simulink model "TType_OffGrid_Inverter_5Step_7Step_SVPWM_THIPWM_Sim"  (R2022b)
settings: Solver=FixedStepDiscrete  StartTime=0.0  StopTime=1  FixedStep=1e-6  RelTol=1e-3
undefined symbols (not defined in the file): L1
libraries: spsSeriesRLCBranchLib x14, spsMosfetLib x12, spsRMSLib x3, simulink x3, spsVoltageMeasurementLib x3, spsThreePhaseVIMeasurementLib x2, spsDCVoltageSourceLib x1, spsGroundLib x1, spsPower3phInstantaneousLib x1, spspowerguiLib x1
settings Model: Creator=XIAO  LastModifiedBy=XIAO
settings SolverCC: AutoInsertRateTranBlk=on
settings DataIOCC: ReturnWorkspaceOutputs=off

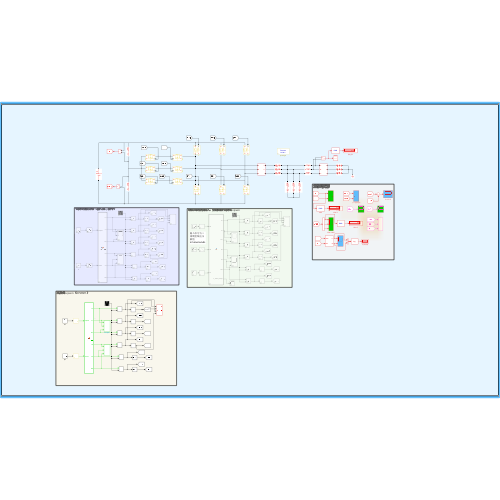
[thumbnail: Simulink's stored preview of the top-level diagram]
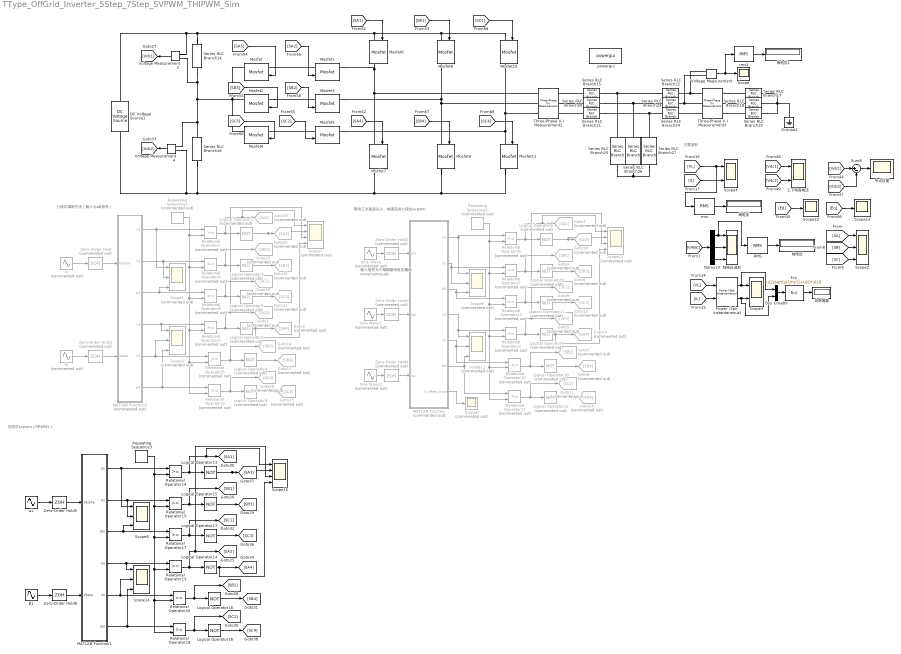
== system TType_OffGrid_Inverter_5Step_7Step_SVPWM_THIPWM_Sim ==
  note: 五段式svpwm（DPWM1）
  note: 输入信号为三相期望线电压幅值
      | m=uinvmx/udc
  note: 等效三次谐波注入，快速完成七段式svpwm
  note: 七段式调制方法（输入为αβ信号）
  note: 主要波形
  Bus Creator : BusCreator  Inputs=2
  DC Voltage Source1 : spsDCVoltageSourceLib/DC Voltage Source  Amplitude=60  Measurements=None
  Demux3 : Demux  Outputs=3
  Fcn : Fcn  Expr=u(1)/sqrt(u(1)*u(1)+u(2)*u(2))
  Goto1 : Goto  Commented=on  GotoTag=SA2
  Goto10 : Goto  Commented=on  GotoTag=SA4
  Goto11 : Goto  Commented=on  GotoTag=SC2
  Goto12 : Goto  Commented=on  GotoTag=SC3
  Goto13 : Goto  Commented=on  GotoTag=SB1
  Goto14 : Goto  Commented=on  GotoTag=SB2
  Goto15 : Goto  Commented=on  GotoTag=SB3
  Goto16 : Goto  Commented=on  GotoTag=SA1
  Goto17 : Goto  Commented=on  GotoTag=SB4
  Goto18 : Goto  Commented=on  GotoTag=SC1
  Goto19 : Goto  Commented=on  GotoTag=SA3
  Goto2 : Goto  Commented=on  GotoTag=SA4
  Goto20 : Goto  Commented=on  GotoTag=SC2
  Goto21 : Goto  Commented=on  GotoTag=SC3
  Goto22 : Goto  Commented=on  GotoTag=SA3
  Goto23 : Goto  Commented=on  GotoTag=SC4
  Goto24 : Goto  Commented=on  GotoTag=SC4
  Goto3 : Goto  Commented=on  GotoTag=SA2
  Goto4 : Goto  Commented=on  GotoTag=SB1
  Goto5 : Goto  Commented=on  GotoTag=SB2
  Goto6 : Goto  Commented=on  GotoTag=SB3
  Goto7 : Goto  Commented=on  GotoTag=SA1
  Goto8 : Goto  Commented=on  GotoTag=SB4
  Goto9 : Goto  Commented=on  GotoTag=SC1
  Ground2 : spsGroundLib/Ground  LConnTagsString=a
  Logical Operator{1..12} (12 alike) : Logic  Commented=on  Operator=NOT  AllPortsSameDT=off  OutDataTypeStr=boolean
  Logical Operator{13..18} (6 alike) : Logic  Operator=NOT  AllPortsSameDT=off  OutDataTypeStr=boolean
  MATLAB Function : MATLAB Function  Commented=on  TreatAsAtomicUnit=on
  MATLAB Function1 : MATLAB Function  TreatAsAtomicUnit=on
  MATLAB Function2 : MATLAB Function  Commented=on  TreatAsAtomicUnit=on
  Mosfet{,1..11} (12 alike) : spsMosfetLib/Mosfet  Ron=0.1  Lon=0  Rd=0.01  Vfd=0  IC=0  Rs=1e5  Cs=inf  Measurements=on
  "Power (3ph, Instantaneous)" : spsPower3phInstantaneousLib/Power (3ph, Instantaneous)
  RMS : spsRMSLib/RMS  TrueRMS=on  Freq=50  RMSInit=120  Ts=1e-6
  Relational Operator{1..12} (12 alike) : RelationalOperator  Commented=on  OutDataTypeStr=boolean  RndMeth=Simplest  InputSameDT=off
  Relational Operator{13..18} (6 alike) : RelationalOperator  OutDataTypeStr=boolean  RndMeth=Simplest  InputSameDT=off
  Repeating Sequence1 : simulink/Sources/Repeating Sequence  Commented=on  rep_seq_t="[0  5e-5  1e-4]"  rep_seq_y=[0 8500 0]
  Repeating Sequence2 : simulink/Sources/Repeating Sequence  Commented=on  rep_seq_t="[0  5e-5  1e-4]"  rep_seq_y=[0 8500 0]
  Repeating Sequence3 : simulink/Sources/Repeating Sequence  rep_seq_t="[0  5e-5  1e-4]"  rep_seq_y=[0 8500 0]
  Scope : Scope
  Scope{1,5,9,11} (4 alike) : Scope  Commented=on  NumInputPorts=3
  Scope10 : Scope
  Scope12 : Scope  Commented=on  NumInputPorts=4
  Scope13 : Scope
  Scope14 : Scope  NumInputPorts=3
  Scope15 : Scope  NumInputPorts=4
  Scope2 : Scope  NumInputPorts=3
  Scope3 : Scope  NumInputPorts=2
  Scope4 : Scope  NumInputPorts=2
  Scope6 : Scope  Commented=on
  Scope7 : Scope  Commented=on  NumInputPorts=4
  Scope8 : Scope  NumInputPorts=3
  Series RLC Branch14 : spsSeriesRLCBranchLib/Series RLC Branch  LConnTagsString=__new0  RConnTagsString=__new0  BranchType=RC  Resistance=0.001  Inductance=1e-3  SetiL0=off  InitialCurrent=0  Capacitance=1000e-6  Setx0=off  InitialVoltage=260  Measurements=None
  Series RLC Branch15 : spsSeriesRLCBranchLib/Series RLC Branch  LConnTagsString=__new0  RConnTagsString=__new0  BranchType=RL  Resistance=1e-3  Inductance=2e-3  SetiL0=off  InitialCurrent=0  Capacitance=5.6e-3  Setx0=off  InitialVoltage=0  Measurements=None
  Series RLC Branch16 : spsSeriesRLCBranchLib/Series RLC Branch  LConnTagsString=__new0  RConnTagsString=__new0  BranchType=RC  Resistance=0.001  Inductance=1e-3  SetiL0=off  InitialCurrent=0  Capacitance=1000e-6  Setx0=off  InitialVoltage=200  Measurements=None
  Series RLC Branch17 : spsSeriesRLCBranchLib/Series RLC Branch  LConnTagsString=__new0  RConnTagsString=__new0  BranchType=RLC  Resistance=200  Inductance=0  SetiL0=off  InitialCurrent=0  Capacitance=0  Setx0=off  InitialVoltage=0  Measurements=None
  Series RLC Branch18 : spsSeriesRLCBranchLib/Series RLC Branch  LConnTagsString=__new0  RConnTagsString=__new0  BranchType=RLC  Resistance=200  Inductance=0  SetiL0=off  InitialCurrent=0  Capacitance=0  Setx0=off  InitialVoltage=0  Measurements=None
  Series RLC Branch19 : spsSeriesRLCBranchLib/Series RLC Branch  LConnTagsString=__new0  RConnTagsString=__new0  BranchType=RLC  Resistance=200  Inductance=0  SetiL0=off  InitialCurrent=0  Capacitance=0  Setx0=off  InitialVoltage=0  Measurements=None
  Series RLC Branch20 : spsSeriesRLCBranchLib/Series RLC Branch  LConnTagsString=__new0  RConnTagsString=__new0  BranchType=RL  Resistance=1e-3  Inductance=2e-3  SetiL0=off  InitialCurrent=0  Capacitance=5.6e-3  Setx0=off  InitialVoltage=0  Measurements=None
  Series RLC Branch21 : spsSeriesRLCBranchLib/Series RLC Branch  LConnTagsString=__new0  RConnTagsString=__new0  BranchType=RL  Resistance=1e-3  Inductance=2e-3  SetiL0=off  InitialCurrent=0  Capacitance=5.6e-3  Setx0=off  InitialVoltage=0  Measurements=None
  Series RLC Branch22 : spsSeriesRLCBranchLib/Series RLC Branch  LConnTagsString=__new0  RConnTagsString=__new0  BranchType=L  Resistance=1e-6  Inductance=1.5e-3  SetiL0=off  InitialCurrent=0  Capacitance=5.6e-3  Setx0=off  InitialVoltage=0  Measurements=None
  Series RLC Branch23 : spsSeriesRLCBranchLib/Series RLC Branch  LConnTagsString=__new0  RConnTagsString=__new0  BranchType=L  Resistance=1e-6  Inductance=1.5e-3  SetiL0=off  InitialCurrent=0  Capacitance=5.6e-3  Setx0=off  InitialVoltage=0  Measurements=None
  Series RLC Branch24 : spsSeriesRLCBranchLib/Series RLC Branch  LConnTagsString=__new0  RConnTagsString=__new0  BranchType=L  Resistance=1e-6  Inductance=1.5e-3  SetiL0=off  InitialCurrent=0  Capacitance=5.6e-3  Setx0=off  InitialVoltage=0  Measurements=None
  Series RLC Branch25 : spsSeriesRLCBranchLib/Series RLC Branch  LConnTagsString=__new0  RConnTagsString=__new0  BranchType=RC  Resistance=3  Inductance=L1  SetiL0=off  InitialCurrent=0  Capacitance=10.5e-6  Setx0=off  InitialVoltage=0  Measurements=None
  Series RLC Branch26 : spsSeriesRLCBranchLib/Series RLC Branch  LConnTagsString=__new0  RConnTagsString=__new0  BranchType=RC  Resistance=3  Inductance=L1  SetiL0=off  InitialCurrent=0  Capacitance=10.5e-6  Setx0=off  InitialVoltage=0  Measurements=None
  Series RLC Branch27 : spsSeriesRLCBranchLib/Series RLC Branch  LConnTagsString=__new0  RConnTagsString=__new0  BranchType=RC  Resistance=3  Inductance=L1  SetiL0=off  InitialCurrent=0  Capacitance=10.5e-6  Setx0=off  InitialVoltage=0  Measurements=None
  Sine Wave : Sin  Commented=on  Amplitude=0.7542  Frequency=2*pi*50  SampleTime=0
  Sine Wave1 : Sin  Commented=on  Amplitude=0.7542  Frequency=2*pi*50  Phase=2*pi/3  SampleTime=0
  Sine Wave2 : Sin  Commented=on  Amplitude=0.7542  Frequency=2*pi*50  Phase=-2*pi/3  SampleTime=0
  Sum8 : Sum  Inputs=|+-
  Three-Phase V-I Measurement2 : spsThreePhaseVIMeasurementLib/Three-Phase V-I Measurement  VoltageMeasurement=phase-to-phase  SetLabelV=on  LabelV=VABC  Vpu=off  VpuLL=off  CurrentMeasurement=yes  SetLabelI=on  LabelI=Iinv  Ipu=off  Pbase=100e6  Vbase=500e3  OutputType=Complex  PhasorSimulation=off  PSBequivalent=0
  Three-Phase V-I Measurement3 : spsThreePhaseVIMeasurementLib/Three-Phase V-I Measurement  VoltageMeasurement=phase-to-ground  SetLabelV=on  LabelV=VL  Vpu=off  VpuLL=off  CurrentMeasurement=yes  SetLabelI=on  LabelI=IL  Ipu=off  Pbase=100e6  Vbase=500e3  OutputType=Complex  PhasorSimulation=off  PSBequivalent=0
  Voltage Measurement : spsVoltageMeasurementLib/Voltage Measurement  PhasorSimulation=off  OutputType=Complex  PSBequivalent=0
  Voltage Measurement2 : spsVoltageMeasurementLib/Voltage Measurement  PhasorSimulation=off  OutputType=Complex  PSBequivalent=0
  Voltage Measurement4 : spsVoltageMeasurementLib/Voltage Measurement  PhasorSimulation=off  OutputType=Complex  PSBequivalent=0
  Zero-Order Hold{,1..4} (5 alike) : ZeroOrderHold  Commented=on  SampleTime=5e-5
  Zero-Order Hold5 : ZeroOrderHold  SampleTime=5e-5
  Zero-Order Hold6 : ZeroOrderHold  SampleTime=5e-5
  powergui : spspowerguiLib/powergui  Priority=1  SimulationMode=Discrete  SampleTime=1e-6  frequency=60  Iterations=50  frequencyindice=0  Pbase=100e6  ErrMax=1e-4  UnitsV=kV  UnitsW=MW  buscounter=0  FunctionMessages=off  echomessages=off  EnableUseOfTLC=off  CurrentSourceSwitches=off  DisableSnubberDevices=off  DisableRonSwitches=off  DisableVfSwitches=off  DisplayEquations=off  AutomaticDiscreteSolvers=off  SolverType=Tustin/Backward Euler (TBE)  Interpol=off  ExternalGateDelay=off  methode=off  Ts=100  x0status=blocks  SPID=on  SwTol=0  HookPort=off  NonlinearTolerance=1e-4  nMaxIteration=100  ContinueOnMaxIteration=off  RestoreLinks=warning  ResistiveCurrentMeasurement=off  Frange=[0:2:500]  Ylog=off  Xlog=on  ShowGrid=off  save=off  variable=ZData  structure=0  ZoomFFT=off  StartTime=0.0  cycles=1  DisplayStyle=1  fundamental=60  FreqAxis=off  MaxFrequency=1000  frequencyindicesteady=1  RmsSteady=1  display=off
  rms : spsRMSLib/RMS  TrueRMS=on  Freq=50  RMSInit=120  Ts=1e-6
  rms1 : spsRMSLib/RMS  TrueRMS=on  Freq=50  RMSInit=120  Ts=1e-6
  α : Sin  Commented=on  Amplitude=26.13  Frequency=100*pi  SampleTime=0
  α1 : Sin  Amplitude=26.13  Frequency=100*pi  SampleTime=0
  β : Sin  Commented=on  Amplitude=26.13  Frequency=100*pi  Phase=pi/2  SampleTime=0
  β1 : Sin  Amplitude=26.13  Frequency=100*pi  Phase=pi/2  SampleTime=0
  上下电容电压 : Scope  NumInputPorts=2
  中点压差 : Scope
  功率因数 : Display
  相电压 : Display
  相电压1 : Display
  线电压 : Display
  线电压波形 : Scope  NumInputPorts=3
  wires:
  Voltage Measurement2/1 -> [Vdc1]
  Voltage Measurement4/1 -> [Vdc2]
  [SA3] -> Mosfet/1
  [SA2] -> Mosfet1/1
  [SB3] -> Mosfet2/1
  [SB2] -> Mosfet3/1
  [SC3] -> Mosfet4/1
  [SC2] -> Mosfet5/1
  [SA1] -> Mosfet6/1
  [SA4] -> Mosfet7/1
  [SB4] -> Mosfet9/1
  [SC4] -> Mosfet11/1
  [SC1] -> Mosfet10/1
  [SB1] -> Mosfet8/1
  β/1 -> Zero-Order Hold1/1
  α/1 -> Zero-Order Hold/1
  Demux3/3 -> 线电压波形/3
  Sum8/1 -> 中点压差/1
  [VL] -> rms/1, Scope4/1
  [IL] -> "Power (3ph, Instantaneous)"/2
  [IL] -> Scope4/2
  "Power (3ph, Instantaneous)"/2 -> Bus Creator/2, Scope3/2
  Bus Creator/1 -> Fcn/1
  Demux3/2 -> 线电压波形/2
  [Ed] -> Scope10/1
  [Vdc1] -> Sum8/1
  [SA] -> Scope2/1
  [Vdc1] -> 上下电容电压/1
  [VL] -> "Power (3ph, Instantaneous)"/1
  [Eq] -> Scope13/1
  Demux3/1 -> RMS/1, 线电压波形/1
  [Vdc2] -> Sum8/2
  [Vdc2] -> 上下电容电压/2
  [SB] -> Scope2/2
  [VABC] -> Demux3/1
  Fcn/1 -> 功率因数/1
  [SC] -> Scope2/3
  "Power (3ph, Instantaneous)"/1 -> Bus Creator/1, Scope3/1
  RMS/1 -> 线电压/1
  rms/1 -> 相电压/1
  Zero-Order Hold/1 -> MATLAB Function2/1(Valpha)
  Zero-Order Hold1/1 -> MATLAB Function2/2(Vbeta)
  Relational Operator2/1 -> Scope7/1, Goto16/1, Logical Operator1/1
  Logical Operator1/1 -> Scope7/2, Goto22/1
  Relational Operator1/1 -> Goto1/1, Scope7/3, Logical Operator2/1
  Logical Operator2/1 -> Goto2/1, Scope7/4
  Logical Operator3/1 -> Goto15/1
  Relational Operator4/1 -> Logical Operator3/1, Goto13/1
  Relational Operator5/1 -> Logical Operator4/1, Goto14/1
  Logical Operator4/1 -> Goto17/1
  Logical Operator8/1 -> Goto23/1
  Logical Operator5/1 -> Goto21/1
  Relational Operator9/1 -> Goto20/1, Logical Operator8/1
  Relational Operator8/1 -> Goto18/1, Logical Operator5/1
  MATLAB Function2/1(U1) -> Scope1/1, Relational Operator2/1
  Repeating Sequence1/1 -> Relational Operator9/2, Relational Operator5/2, Relational Operator1/2, Relational Operator8/2, Relational Operator4/2, Relational Operator2/2
  MATLAB Function2/3(W1) -> Scope1/3, Relational Operator8/1
  MATLAB Function2/2(V1) -> Scope1/2, Relational Operator4/1
  MATLAB Function2/4(U2) -> Scope5/1, Relational Operator1/1
  MATLAB Function2/5(V2) -> Relational Operator5/1, Scope5/2
  MATLAB Function2/6(W2) -> Relational Operator9/1, Scope5/3
  Voltage Measurement/1 -> rms1/1, Scope/1
  rms1/1 -> 相电压1/1
  Sine Wave/1 -> Zero-Order Hold2/1
  Sine Wave2/1 -> Zero-Order Hold4/1
  Sine Wave1/1 -> Zero-Order Hold3/1
  Zero-Order Hold2/1 -> MATLAB Function/1(tsa)
  Zero-Order Hold3/1 -> MATLAB Function/2(tsb)
  Zero-Order Hold4/1 -> MATLAB Function/3(tsc)
  Logical Operator11/1 -> Goto12/1
  Relational Operator6/1 -> Scope12/1, Goto7/1, Logical Operator6/1
  MATLAB Function/5(V2) -> Relational Operator10/1, Scope11/2
  MATLAB Function/4(U2) -> Scope11/1, Relational Operator3/1
  Relational Operator11/1 -> Goto9/1, Logical Operator11/1
  Repeating Sequence2/1 -> Relational Operator12/2, Relational Operator10/2, Relational Operator3/2, Relational Operator11/2, Relational Operator7/2, Relational Operator6/2
  MATLAB Function/3(W1) -> Relational Operator11/1, Scope9/3
  Relational Operator12/1 -> Goto11/1, Logical Operator12/1
  MATLAB Function/6(W2) -> Relational Operator12/1, Scope11/3
  Logical Operator9/1 -> Goto6/1
  MATLAB Function/1(U1) -> Relational Operator6/1, Scope9/1
  Logical Operator7/1 -> Goto10/1, Scope12/4
  Relational Operator10/1 -> Logical Operator10/1, Goto5/1
  Relational Operator7/1 -> Logical Operator9/1, Goto4/1
  Logical Operator10/1 -> Goto8/1
  Logical Operator6/1 -> Scope12/2, Goto19/1
  Relational Operator3/1 -> Goto3/1, Scope12/3, Logical Operator7/1
  Logical Operator12/1 -> Goto24/1
  MATLAB Function/2(V1) -> Scope9/2, Relational Operator7/1
  MATLAB Function/7(V_offset_scope) -> Scope6/1
  Relational Operator14/1 -> Scope15/1, [SA1], Logical Operator13/1
  Zero-Order Hold5/1 -> MATLAB Function1/1(Valpha)
  MATLAB Function1/5(V2) -> Relational Operator16/1, Scope14/2
  Logical Operator17/1 -> [SC3]
  MATLAB Function1/2(V1) -> Scope8/2, Relational Operator15/1
  Relational Operator17/1 -> [SC1], Logical Operator17/1
  Repeating Sequence3/1 -> Relational Operator18/2, Relational Operator16/2, Relational Operator13/2, Relational Operator17/2, Relational Operator15/2, Relational Operator14/2
  Zero-Order Hold6/1 -> MATLAB Function1/2(Vbeta)
  Relational Operator18/1 -> [SC2], Logical Operator18/1
  MATLAB Function1/3(W1) -> Scope8/3, Relational Operator17/1
  Logical Operator15/1 -> [SB3]
  MATLAB Function1/1(U1) -> Scope8/1, Relational Operator14/1
  Logical Operator14/1 -> [SA4], Scope15/4
  Relational Operator16/1 -> Logical Operator16/1, [SB2]
  Relational Operator15/1 -> Logical Operator15/1, [SB1]
  MATLAB Function1/6(W2) -> Relational Operator18/1, Scope14/3
  MATLAB Function1/4(U2) -> Scope14/1, Relational Operator13/1
  Logical Operator13/1 -> Scope15/2, [SA3]
  Logical Operator16/1 -> [SB4]
  Relational Operator13/1 -> [SA2], Scope15/3, Logical Operator14/1
  Logical Operator18/1 -> [SC4]
  β1/1 -> Zero-Order Hold6/1
  α1/1 -> Zero-Order Hold5/1
  connections:
  Series RLC Branch16/LConn1 -- Voltage Measurement2/LConn2 -- Series RLC Branch14/RConn1 -- Mosfet/RConn1 -- Mosfet2/RConn1 -- Mosfet4/RConn1 -- Voltage Measurement4/LConn1
  Series RLC Branch16/RConn1 -- Mosfet11/RConn1 -- Mosfet9/RConn1 -- Mosfet7/RConn1 -- DC Voltage Source1/LConn1 -- Voltage Measurement4/LConn2
  Series RLC Branch14/LConn1 -- Mosfet10/LConn1 -- Mosfet8/LConn1 -- Mosfet6/LConn1 -- DC Voltage Source1/RConn1 -- Voltage Measurement2/LConn1
  Mosfet/LConn1 -- Mosfet1/LConn1
  Mosfet2/LConn1 -- Mosfet3/LConn1
  Mosfet4/LConn1 -- Mosfet5/LConn1
  Mosfet7/LConn1 -- Mosfet1/RConn1 -- Mosfet6/RConn1 -- Three-Phase V-I Measurement2/LConn1
  Mosfet8/RConn1 -- Mosfet9/LConn1 -- Three-Phase V-I Measurement2/LConn2 -- Mosfet3/RConn1
  Mosfet11/LConn1 -- Three-Phase V-I Measurement2/LConn3 -- Mosfet10/RConn1 -- Mosfet5/RConn1
  Series RLC Branch27/RConn1 -- Series RLC Branch26/RConn1 -- Series RLC Branch25/RConn1
  Series RLC Branch26/LConn1 -- Series RLC Branch20/RConn1 -- Series RLC Branch23/LConn1
  Series RLC Branch22/LConn1 -- Series RLC Branch25/LConn1 -- Series RLC Branch15/RConn1
  Series RLC Branch18/RConn1 -- Series RLC Branch19/RConn1 -- Series RLC Branch17/RConn1 -- Ground2/LConn1
  Series RLC Branch27/LConn1 -- Series RLC Branch21/RConn1 -- Series RLC Branch24/LConn1
  Three-Phase V-I Measurement3/LConn1 -- Voltage Measurement/LConn1 -- Series RLC Branch22/RConn1
  Series RLC Branch15/LConn1 -- Three-Phase V-I Measurement2/RConn1
  Series RLC Branch20/LConn1 -- Three-Phase V-I Measurement2/RConn2
  Three-Phase V-I Measurement3/LConn3 -- Series RLC Branch24/RConn1
  Three-Phase V-I Measurement3/LConn2 -- Voltage Measurement/LConn2 -- Series RLC Branch23/RConn1
  Series RLC Branch21/LConn1 -- Three-Phase V-I Measurement2/RConn3
  Three-Phase V-I Measurement3/RConn1 -- Series RLC Branch17/LConn1
  Series RLC Branch19/LConn1 -- Three-Phase V-I Measurement3/RConn3
  Three-Phase V-I Measurement3/RConn2 -- Series RLC Branch18/LConn1

== matlab function TType_OffGrid_Inverter_5Step_7Step_SVPWM_THIPWM_Sim/MATLAB Function ==
  data: tsa input; U1 output; tsb input; tsc input; V1 output; W1 output; U2 output; V2 output; W2 output; V_offset_scope output
function [U1, V1, W1, U2, V2, W2, V_offset_scope] = fcn(tsa, tsb, tsc)
%#codegen
% =========================================================================
% 功能: 简化版载波等效三电平SVPWM算法（含三次谐波可视化输出端口）
% 输入: tsa, tsb, tsc —— 三相标准正弦波信号（幅值代表调制比 m）
% 输出: 
%   U1, V1, W1: 范围在 -8500 ~ 8500 的标准基准调制波
%   U2, V2, W2: 范围在 0 ~ 17000 的抬升调制波
%   V_offset_scope: 缩放到定时器计数域的三次谐波波形 (范围约 +/-1700)
% =========================================================================

%% 1. 定义系统常数与硬件计数周期
ARR = 8500; % 半个开关周期计数值（对应单三角载波峰值）

% k 为调制比缩放系数，此处使用你代码中提供的 1.1547 (2/sqrt(3))
% 注意：使用该系数且输入幅值为 0.7542 时，最终物理线电压有效值为 32VRMS。
k = 1/0.866;  

%% 2. 基准缩放 (对应图中的 K- 模块)
va = k * tsa;
vb = k * tsb;
vc = k * tsc;

%% 3. 逻辑归一化（对应图中 Switch 模块逻辑）
if va > 0
    ya = va;
else
    ya = va + 1.0;
end

if vb > 0
    yb = vb;
else
    yb = vb + 1.0;
end

if vc > 0
    yc = vc;
else
    yc = vc + 1.0;
end

%% 4. 寻找虚拟空间的最值
y_max = max([ya, yb, yc]);
y_min = min([ya, yb, yc]);

%% 5. 三次谐波/零序分量注入计算 (Normalized)
v_offset = 0.5 * (1.0 - y_max - y_min);

%% 6. 合成基础归一化羊角波（此时范围严格在 [-1, 1] 空间内）
sa_norm = va + v_offset;
sb_norm = vb + v_offset;
sc_norm = vc + v_offset;

%% 7. 硬件计数域缩放与双波复制
% 放大到定时器半周期计数值域 [-8500, 8500]
U1 = sa_norm * double(ARR);
V1 = sb_norm * double(ARR);
W1 = sc_norm * double(ARR);

% 整体向上抬升一个 ARR，范围变为 [0, 17000]
U2 = U1 + double(ARR);
V2 = V1 + double(ARR);
W2 = W1 + double(ARR);

%% 8. 【新增】将三次谐波波形也放大到硬件计数域，用于在 Scope 中清晰观察
V_offset_scope = v_offset * double(ARR);

end

== matlab function TType_OffGrid_Inverter_5Step_7Step_SVPWM_THIPWM_Sim/MATLAB Function2 ==
  data: Valpha input; U1 output; Vbeta input; V1 output; W1 output; U2 output; V2 output; W2 output
function [U1, V1, W1, U2, V2, W2] = svpwm_3level_paper_verify(Valpha, Vbeta)
% #codegen
% =========================================================================
% 功能: 结构优化版三电平NPC逆变器SVPWM算法（单载波双调制波输出版）
% 架构说明: 仿照标准两电平七段式结构重构。
% 输出说明:
%   U1, V1, W1: 范围在 -8500 ~ 8500 的标准基准调制波（用于控制外侧管 S1）
%   U2, V2, W2: 范围在 0 ~ 17000 的抬升调制波（用于控制内侧管 S2）
% 硬件映射: 配合一组 0 ~ 8500 的三角载波，即可直接跑通三电平NPC的4路互补PWM。
% =========================================================================

%% 1. 定义系统常数
Udc   = 60;              % 直流母线电压
ARR   = 8500;            % 半个开关周期计数值（完整周期2*ARR）
sqrt3 = 1.732050807568877;

%% ================== 第一步：大扇区判断 (N因子法) ==================
A = Vbeta;
B = (sqrt3/2) * Valpha - 0.5 * Vbeta;
C = -(sqrt3/2) * Valpha - 0.5 * Vbeta;

a = double(A > 0);
b = double(B > 0);
c = double(C > 0);
N = a + 2*b + 4*c;

sector_map = [2, 6, 1, 4, 3, 5]; 
S_big = sector_map(N);

%% ================== 第二步：小扇区判断 (空间旋转与直线方程) ==================
theta_global = atan2(Vbeta, Valpha);
if theta_global < 0
    theta_global = theta_global + 2*pi;
end

% 空间对称旋转，收敛至第一大扇区 [0, pi/3]
theta1 = theta_global - double(S_big - 1) * (pi/3);

Vamp = sqrt(Valpha^2 + Vbeta^2);
Valpha1 = Vamp * cos(theta1);
Vbeta1 = Vamp * sin(theta1);

% 执行二叉决策树判定小扇区（与论文图4-7完全一致）
if theta1 >= pi/6
    if (Vbeta1 - (sqrt3/6)*Udc) >= 0
        S_small = 6; 
    else
        if (-sqrt3*Valpha1 - Vbeta1 + (sqrt3/3)*Udc) >= 0
            S_small = 2; 
        else
            S_small = 4; 
        end
    end
else
    if (sqrt3*Valpha1 - Vbeta1 - (sqrt3/3)*Udc) >= 0
        S_small = 5; 
    else
        if (-sqrt3*Valpha1 - Vbeta1 + (sqrt3/3)*Udc) >= 0
            S_small = 1; 
        else
            S_small = 3; 
        end
    end
end

%% ================== 第三步：合成矢量时间计算 ==================
m = (sqrt3 * Vamp) / Udc;
m = min(m, 1.1547); % 三电平SVPWM最大线性调制比
Ta = 0; Tb = 0; Tc = 0;

switch S_small
    case {1, 2} % 对应论文公式 (4-17)
        Ta = 2 * m * ARR * sin(theta1);
        Tb = ARR - 2 * m * ARR * sin(pi/3 + theta1);
        Tc = 2 * m * ARR * sin(pi/3 - theta1);
        
    case {3, 4} % 对应论文公式 (4-20)
        Ta = ARR - 2 * m * ARR * sin(theta1);
        Tb = -ARR + 2 * m * ARR * sin(pi/3 + theta1);
        Tc = ARR - 2 * m * ARR * sin(pi/3 - theta1);
        
    case 5 % 对应论文公式 (4-22)
        Ta = 2 * m * ARR * sin(theta1);
        Tb = 2 * ARR - 2 * m * ARR * sin(pi/3 + theta1);
        Tc = -ARR + 2 * m * ARR * sin(pi/3 - theta1);
        
    case 6 % 对应论文公式 (4-24)
        Ta = -ARR + 2 * m * ARR * sin(theta1);
        Tb = 2 * ARR - 2 * m * ARR * sin(pi/3 + theta1);
        Tc = 2 * m * ARR * sin(pi/3 - theta1);
end

%% ================== 第四步：工程过调制保护与限幅 ==================
if Ta < 0, Ta = 0; end
if Tb < 0, Tb = 0; end
if Tc < 0, Tc = 0; end

Tsum = Ta + Tb + Tc;
if Tsum > ARR
    scale = ARR / Tsum;
    Ta = Ta * scale;
    Tb = Tb * scale;
    Tc = Tc * scale;
end

%% ================== 第五步：直观的基础调制分量计算 (高/中/低需求) ==================
m_high = 0; m_mid = 0; m_low = 0;

if mod(S_big, 2) ~= 0
    % ----------------- 奇数大扇区时的时间分配 -----------------
    switch S_small
        case 1
            m_high = (Tc/2) / ARR;
            m_mid  = (-Tc/2) / ARR;
            m_low  = (-Tc/2 - Ta) / ARR;
        case 2
            m_high = (Tc + Ta/2) / ARR;
            m_mid  = (Ta/2) / ARR;
            m_low  = (-Ta/2) / ARR;
        case 3
            m_high = (Tb + Ta/2) / ARR;
            m_mid  = (-Ta/2) / ARR;
            m_low  = -(ARR - Ta/2) / ARR;
        case 4
            m_high = (ARR - Tc/2) / ARR;
            m_mid  = (Tc/2) / ARR;
            m_low  = (-Tc/2 - Tb) / ARR;
        case 5
            m_high = (ARR - Tb/2) / ARR;
            m_mid  = (-Tb/2 - Tc) / ARR;  
            m_low  = -(ARR - Tb/2) / ARR;
        case 6
            m_high = (ARR - Tb/2) / ARR;
            m_mid  = (Ta + Tb/2) / ARR;
            m_low  = -(ARR - Tb/2) / ARR;
    end
else
    % ----------------- 偶数大扇区时的时间分配 -----------------
    switch S_small
        case 1
            m_high = (Ta + Tc/2) / ARR;    
            m_mid  = (Tc/2) / ARR;         
            m_low  = (-Tc/2) / ARR;        
        case 2
            m_high = (Ta/2) / ARR;
            m_mid  = (-Ta/2) / ARR;
            m_low  = (-Ta/2 - Tc) / ARR;
        case 3
            m_high = (ARR - Ta/2) / ARR;
            m_mid  = (Ta/2) / ARR;
            m_low  = (-Ta/2 - Tb) / ARR;  
        case 4
            m_high = (Tb + Tc/2) / ARR;
            m_mid  = (-Tc/2) / ARR;
            m_low  = -(ARR - Tc/2) / ARR;
        case 5
            m_high = (ARR - Tb/2) / ARR;
            m_mid  = (Tc + Tb/2) / ARR;
            m_low  = -(ARR - Tb/2) / ARR;
        case 6
            m_high = (ARR - Tb/2) / ARR;
            m_mid  = (-Ta - Tb/2) / ARR;
            m_low  = -(ARR - Tb/2) / ARR;
    end
end

%% ================== 第六步：物理三相直接映射 (归一化 [-1,1]) ==================
U_norm = 0; V_norm = 0; W_norm = 0;
switch S_big
    case 1  % 大扇区1: A > B > C
        U_norm = m_high;  V_norm = m_mid;   W_norm = m_low;
    case 2  % 大扇区2: B > A > C
        U_norm = m_mid;   V_norm = m_high;  W_norm = m_low;
    case 3  % 大扇区3: B > C > A
        U_norm = m_low;   V_norm = m_high;  W_norm = m_mid;
    case 4  % 大扇区4: C > B > A
        U_norm = m_low;   V_norm = m_mid;   W_norm = m_high;
    case 5  % 大扇区5: C > A > B
        U_norm = m_mid;   V_norm = m_low;   W_norm = m_high;
    case 6  % 大扇区6: A > C > B
        U_norm = m_high;  V_norm = m_low;   W_norm = m_mid;
end

%% ================== 第七步：【新增】硬件计数域缩放与双波复制 ==================
% 1. 第一组调制波：直接放大到定时器半周期计数值域 [-8500, 8500]
U1 = U_norm * double(ARR);
V1 = V_norm * double(ARR);
W1 = W_norm * double(ARR);

% 2. 第二组调制波：在第一组的基础上整体向上抬升一个 ARR，范围变为 [0, 17000]
U2 = U1 + double(ARR);
V2 = V1 + double(ARR);
W2 = W1 + double(ARR);

end

== matlab function TType_OffGrid_Inverter_5Step_7Step_SVPWM_THIPWM_Sim/MATLAB Function1 ==
  data: Valpha input; U1 output; Vbeta input; V1 output; W1 output; U2 output; V2 output; W2 output
function [U1, V1, W1, U2, V2, W2] = svpwm_3level_paper_verify(Valpha, Vbeta)
% #codegen
% =========================================================================
% 功能: 结构优化版三电平NPC逆变器五段式SVPWM算法（DPWM1 调制版）
% 架构说明: 在标准七段式基础上注入动态零序电压，完美实现论文表4-4的五段式发波逻辑。
% 输出说明:
%   U1, V1, W1: 范围在 -8500 ~ 8500 的标准基准调制波（用于控制外侧管 S1）
%   U2, V2, W2: 范围在 0 ~ 17000 的抬升调制波（用于控制内侧管 S2）
% 硬件映射: 配合一组 0 ~ 8500 的三角载波，即可直接跑通三电平NPC的4路互补PWM。
% =========================================================================
%% 1. 定义系统常数
Udc   = 60;              % 直流母线电压
ARR   = 8500;            % 半个开关周期计数值（完整周期2*ARR）
sqrt3 = 1.732050807568877;

%% ================== 第一步：大扇区判断 (N因子法) ==================
A = Vbeta;
B = (sqrt3/2) * Valpha - 0.5 * Vbeta;
C = -(sqrt3/2) * Valpha - 0.5 * Vbeta;
a = double(A > 0);
b = double(B > 0);
c = double(C > 0);
N = a + 2*b + 4*c;
sector_map = [2, 6, 1, 4, 3, 5]; 
S_big = sector_map(N);

%% ================== 第二步：小扇区判断 (空间旋转与直线方程) ==================
theta_global = atan2(Vbeta, Valpha);
if theta_global < 0
    theta_global = theta_global + 2*pi;
end
% 空间对称旋转，收敛至第一大扇区 [0, pi/3]
theta1 = theta_global - double(S_big - 1) * (pi/3);
Vamp = sqrt(Valpha^2 + Vbeta^2);
Valpha1 = Vamp * cos(theta1);
Vbeta1 = Vamp * sin(theta1);

% 执行二叉决策树判定小扇区（与论文图4-7完全一致）
if theta1 >= pi/6
    if (Vbeta1 - (sqrt3/6)*Udc) >= 0
        S_small = 6; 
    else
        if (-sqrt3*Valpha1 - Vbeta1 + (sqrt3/3)*Udc) >= 0
            S_small = 2; 
        else
            S_small = 4; 
        end
    end
else
    if (sqrt3*Valpha1 - Vbeta1 - (sqrt3/3)*Udc) >= 0
        S_small = 5; 
    else
        if (-sqrt3*Valpha1 - Vbeta1 + (sqrt3/3)*Udc) >= 0
            S_small = 1; 
        else
            S_small = 3; 
        end
    end
end

%% ================== 第三步：合成矢量时间计算 ==================
m = (sqrt3 * Vamp) / Udc;
m = min(m, 1.1547); % 三电平SVPWM最大线性调制比
Ta = 0; Tb = 0; Tc = 0;
switch S_small
    case {1, 2} % 对应论文公式 (4-17)
        Ta = 2 * m * ARR * sin(theta1);
        Tb = ARR - 2 * m * ARR * sin(pi/3 + theta1);
        Tc = 2 * m * ARR * sin(pi/3 - theta1);
        
    case {3, 4} % 对应论文公式 (4-20)
        Ta = ARR - 2 * m * ARR * sin(theta1);
        Tb = -ARR + 2 * m * ARR * sin(pi/3 + theta1);
        Tc = ARR - 2 * m * ARR * sin(pi/3 - theta1);
        
    case 5 % 对应论文公式 (4-22)
        Ta = 2 * m * ARR * sin(theta1);
        Tb = 2 * ARR - 2 * m * ARR * sin(pi/3 + theta1);
        Tc = -ARR + 2 * m * ARR * sin(pi/3 - theta1);
        
    case 6 % 对应论文公式 (4-24)
        Ta = -ARR + 2 * m * ARR * sin(theta1);
        Tb = 2 * ARR - 2 * m * ARR * sin(pi/3 + theta1);
        Tc = 2 * m * ARR * sin(pi/3 - theta1);
end

%% ================== 第四步：工程过调制保护与限幅 ==================
if Ta < 0, Ta = 0; end
if Tb < 0, Tb = 0; end
if Tc < 0, Tc = 0; end
Tsum = Ta + Tb + Tc;
if Tsum > ARR
    scale = ARR / Tsum;
    Ta = Ta * scale;
    Tb = Tb * scale;
    Tc = Tc * scale;
end

%% ================== 第五步：直观的基础调制分量计算 (七段式基准) ==================
m_high = 0; m_mid = 0; m_low = 0;
if mod(S_big, 2) ~= 0
    % ----------------- 奇数大扇区时的时间分配 -----------------
    switch S_small
        case 1
            m_high = (Tc/2) / ARR;
            m_mid  = (-Tc/2) / ARR;
            m_low  = (-Tc/2 - Ta) / ARR;
        case 2
            m_high = (Tc + Ta/2) / ARR;
            m_mid  = (Ta/2) / ARR;
            m_low  = (-Ta/2) / ARR;
        case 3
            m_high = (Tb + Ta/2) / ARR;
            m_mid  = (-Ta/2) / ARR;
            m_low  = -(ARR - Ta/2) / ARR;
        case 4
            m_high = (ARR - Tc/2) / ARR;
            m_mid  = (Tc/2) / ARR;
            m_low  = (-Tc/2 - Tb) / ARR;
        case 5
            m_high = (ARR - Tb/2) / ARR;
            m_mid  = (-Tb/2 - Tc) / ARR;  
            m_low  = -(ARR - Tb/2) / ARR;
        case 6
            m_high = (ARR - Tb/2) / ARR;
            m_mid  = (Ta + Tb/2) / ARR;
            m_low  = -(ARR - Tb/2) / ARR;
    end
else
    % ----------------- 偶数大扇区时的时间分配 -----------------
    switch S_small
        case 1
            m_high = (Ta + Tc/2) / ARR;    
            m_mid  = (Tc/2) / ARR;         
            m_low  = (-Tc/2) / ARR;        
        case 2
            m_high = (Ta/2) / ARR;
            m_mid  = (-Ta/2) / ARR;
            m_low  = (-Ta/2 - Tc) / ARR;
        case 3
            m_high = (ARR - Ta/2) / ARR;
            m_mid  = (Ta/2) / ARR;
            m_low  = (-Ta/2 - Tb) / ARR;  
        case 4
            m_high = (Tb + Tc/2) / ARR;
            m_mid  = (-Tc/2) / ARR;
            m_low  = -(ARR - Tc/2) / ARR;
        case 5
            m_high = (ARR - Tb/2) / ARR;
            m_mid  = (Tc + Tb/2) / ARR;
            m_low  = -(ARR - Tb/2) / ARR;
        case 6
            m_high = (ARR - Tb/2) / ARR;
            m_mid  = (-Ta - Tb/2) / ARR;
            m_low  = -(ARR - Tb/2) / ARR;
    end
end

%% ================== 【新增】第五步b：DPWM1 五段式调制优化层 ==================
% 根据小扇区特征注入动态零序偏置，实现某一相全程不动作
k_dpwm = 0;
switch S_small
    case {1, 2} 
        % 对应论文表4-4中的 A、B 小扇区（内侧区域）
        % 核心逻辑：中相（m_mid）钳位至零点（中点电平O），使其开关完全不切换
        k_dpwm = 0.0 - m_mid;
        
    case {3, 5} 
        % 对应论文表4-4中的 C 小扇区（外侧右强相区域）
        % 核心逻辑：高相（m_high）钳位至正母线（P电平，归一化值为1.0）
        k_dpwm = 1.0 - m_high;
        
    case {4, 6} 
        % 对应论文表4-4中的 D 小扇区（外侧左强相区域）
        % 核心逻辑：低相（m_low）钳位至负母线（N电平，归一化值为-1.0）
        k_dpwm = -1.0 - m_low;
end

% 动态注入零序分量，转化为五段式不连续发波波形
m_high = m_high + k_dpwm;
m_mid  = m_mid  + k_dpwm;
m_low  = m_low  + k_dpwm;

%% ================== 第六步：物理三相直接映射 (归一化 [-1,1]) ==================
U_norm = 0; V_norm = 0; W_norm = 0;
switch S_big
    case 1  % 大扇区1: A > B > C
        U_norm = m_high;  V_norm = m_mid;   W_norm = m_low;
    case 2  % 大扇区2: B > A > C
        U_norm = m_mid;   V_norm = m_high;  W_norm = m_low;
    case 3  % 大扇区3: B > C > A
        U_norm = m_low;   V_norm = m_high;  W_norm = m_mid;
    case 4  % 大扇区4: C > B > A
        U_norm = m_low;   V_norm = m_mid;   W_norm = m_high;
    case 5  % 大扇区5: C > A > B
        U_norm = m_mid;   V_norm = m_low;   W_norm = m_high;
    case 6  % 大扇区6: A > C > B
        U_norm = m_high;  V_norm = m_low;   W_norm = m_mid;
end

%% ================== 第七步：硬件计数域缩放与双波复制 ==================
% 1. 第一组调制波：直接放大到定时器半周期计数值域 [-8500, 8500]
U1 = U_norm * double(ARR);
V1 = V_norm * double(ARR);
W1 = W_norm * double(ARR);

% 2. 第二组调制波：在第一组的基础上整体向上抬升一个 ARR，范围变为 [0, 17000]
U2 = U1 + double(ARR);
V2 = V1 + double(ARR);
W2 = W1 + double(ARR);
end
